simulink model "mdldrkozpo"  (Simulink 7.8)
settings: Solver=ode45  StartTime=0.0  StopTime=10.0  RelTol=1e-3
settings Model: Creator=klempond  LastModifiedBy=polacekm
settings GRTTargetCC: CombineOutputUpdateFcns=on

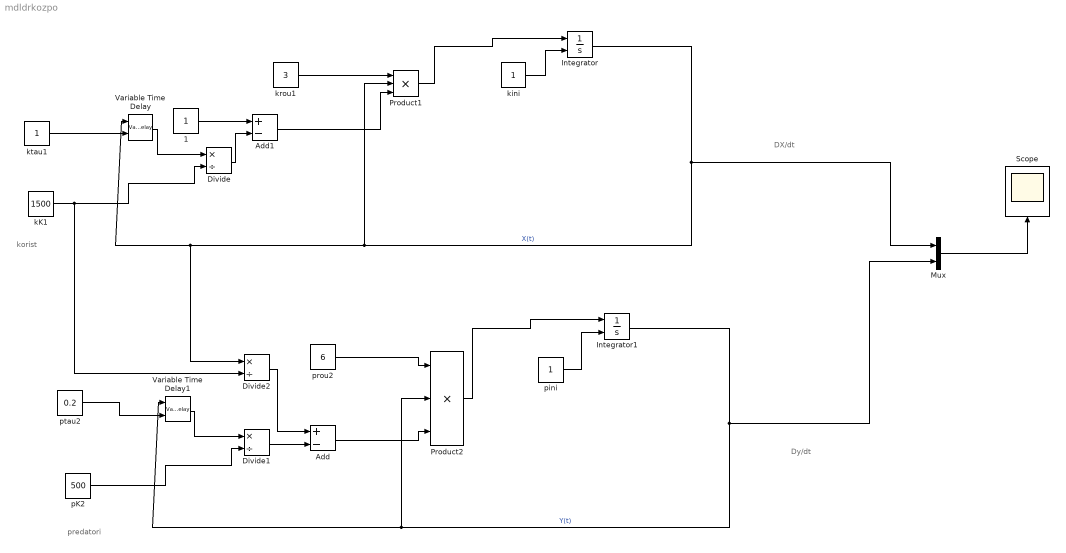
== system mdldrkozpo ==
  note: DX/dt
  note: Dy/dt
  note: korist
  note: predatori
  1 : Constant
  Add : Sum  Inputs=+-
  Add1 : Sum  Inputs=+-
  Divide : Product  Inputs=*/
  Divide1 : Product  Inputs=*/
  Divide2 : Product  Inputs=*/
  Integrator : Integrator  InitialConditionSource=external  InitialCondition=10
  Integrator1 : Integrator  InitialConditionSource=external  InitialCondition=10
  Mux : Mux  Inputs=2
  Product1 : Product  Inputs=3  RndMeth=Zero
  Product2 : Product  Inputs=3  RndMeth=Zero
  Scope : Scope
      settings: YMin=-1e+134  YMax=1.6e+135  SaveName=sc
  Variable Time Delay : VariableTransportDelay  MaximumDelay=10
  Variable Time Delay1 : VariableTransportDelay  MaximumDelay=10
  kK1 : Constant  Value=1500
  kini : Constant
  krou1 : Constant  Value=3
  ktau1 : Constant
  pK2 : Constant  Value=500
  pini : Constant
  prou2 : Constant  Value=6
  ptau2 : Constant  Value=0.2
  wires:
  krou1/1 -> Product1/1
  Product1/1 -> Integrator/1
  Variable Time Delay/1 -> Divide/1
  kK1/1 -> Divide/2, Divide2/2
  1/1 -> Add1/1
  Integrator/1 -> Product1/2, Divide2/1, Variable Time Delay/1, Mux/1  "X(t)"
  prou2/1 -> Product2/1
  Product2/1 -> Integrator1/1
  Variable Time Delay1/1 -> Divide1/1
  pK2/1 -> Divide1/2
  Divide1/1 -> Add/2
  Integrator1/1 -> Mux/2, Product2/2, Variable Time Delay1/1  "Y(t)"
  Divide2/1 -> Add/1
  Mux/1 -> Scope/1
  Add/1 -> Product2/3
  Add1/1 -> Product1/3
  Divide/1 -> Add1/2
  ktau1/1 -> Variable Time Delay/2
  ptau2/1 -> Variable Time Delay1/2
  kini/1 -> Integrator/2
  pini/1 -> Integrator1/2
